simulink model "SIM_NonlinearPIwAW_2017b"  (R2017b)
settings: Solver=FixedStepAuto  StartTime=0.0  StopTime=9*0.25  FixedStep=h  RelTol=1e-3
values from neighbouring files (symbols this model uses):
  h = 1e-5    (= 1e-05)    [init.m]
  J = [0 -1; 1 0]    [generate_EKF.m]    (also in init.m)
  log_ts = 1e-5    (= 1e-05)    [init.m]
  lut_fr =     [friction.mat]
  omegam_ref = 157    [init.m]
  p = 2    [generate_EKF.m]
  P_init_dist = W_dist_noise    [init.m]
  pmsm_sew =     [config.mat]
  Psi_jac = [0.121, 0; 0, 0.0769]    [init.m]
  rsm_za =     [config.mat]
  SysConfig_SamplingTimeA = 0.00025    [config.mat]
  SysConfig_SamplingTimeB = 0.00025    [config.mat]
  u_DC = 556    [init.m]
  V_dist_noise = diag([2e0, 2e0])    [init.m]
  W_dist_noise = diag([1e-2, 1e-2, 1e4, 1e4])    [init.m]
  x_e_init_dist = zeros(4,1)    [init.m]
undefined symbols (not defined in the file or in its folder): DiscIntNeverNeededParam, f_pwm, k_i, k_p_tilde, uhat
libraries: simulink x4
(part 2 of 2)

== system SIM_NonlinearPIwAW_2017b/RSM_Control/Linear MPC/steady-state input computation ==
  psisk_ref : Inport
  wk : Inport  Port=2
  dist_est : Inport  Port=3
  Gain3 : Gain  Gain=J  Multiplication=Matrix(K*u)
  Gain4 : Gain  Gain=rsm_za.Rs
  Matrix Multiply : Product  Multiplication=Matrix(*)
  Product1 : Product
  Sum3 : Sum  Inputs=|++
  Sum4 : Sum  Inputs=|+-
  Unit Delay1 : UnitDelay  InitialCondition=[0,0]  SampleTime=-1
  Unit Delay2 : UnitDelay  InitialCondition=[0]  SampleTime=-1
  Unit Delay3 : UnitDelay  InitialCondition=[0,0]  SampleTime=-1
  inverse of dPsi/di : Constant  Value=inv(Psi_jac)
  u_ref : Outport
  wires:
  Sum3/1 -> u_ref/1
  dist_est/1 -> Unit Delay3/1
  Gain3/1 -> Product1/1
  psisk_ref/1 -> Gain3/1, Unit Delay1/1
  wk/1 -> Unit Delay2/1
  Matrix Multiply/1 -> Gain4/1
  Sum4/1 -> Sum3/2
  Gain4/1 -> Sum4/1
  Product1/1 -> Sum3/1
  Unit Delay1/1 -> Matrix Multiply/2
  Unit Delay2/1 -> Product1/2
  Unit Delay3/1 -> Sum4/2
  inverse of dPsi/di/1 -> Matrix Multiply/1

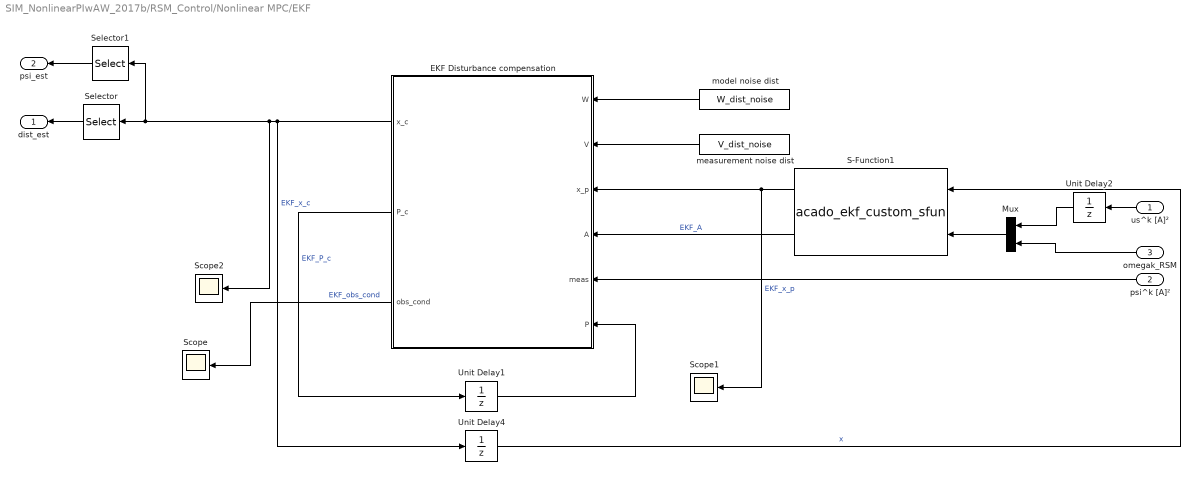
== system SIM_NonlinearPIwAW_2017b/RSM_Control/Nonlinear MPC/EKF  ==
  us^k [A]² : Inport
  psi^k [A]² : Inport  Port=2
  omegak_RSM : Inport  Port=3
  EKF Disturbance compensation : MATLAB Function  TreatAsAtomicUnit=on
  Mux : Mux  Inputs=2
  S-Function1 : S-Function  FunctionName=acado_ekf_custom_sfun  Parameters=[0 0 0 0]  SFunctionDeploymentMode=off  EnableBusSupport=off
  Scope : Scope
  Scope1 : Scope
  Scope2 : Scope
  Selector : Selector  InputPortWidth=4  IndexOptions=Index vector (dialog)  Indices=[3 4]  OutputSizes=1
  Selector1 : Selector  InputPortWidth=4  IndexOptions=Index vector (dialog)  Indices=[1 2]  OutputSizes=1
  Unit Delay1 : UnitDelay  InitialCondition=P_init_dist  SampleTime=-1
  Unit Delay2 : UnitDelay  InitialCondition=[0,0]  SampleTime=-1
  Unit Delay4 : UnitDelay  InitialCondition=x_e_init_dist  SampleTime=-1
  measurement noise dist : Constant  Value=V_dist_noise
  model noise dist : Constant  Value=W_dist_noise
  dist_est : Outport
  psi_est : Outport  Port=2
  wires:
  EKF Disturbance compensation/2(P_c) -> Unit Delay1/1  "EKF_P_c"
  measurement noise dist/1 -> EKF Disturbance compensation/2(V)
  EKF Disturbance compensation/3(obs_cond) -> Scope/1  "EKF_obs_cond"
  model noise dist/1 -> EKF Disturbance compensation/1(W)
  Unit Delay4/1 -> S-Function1/1  "x"
  EKF Disturbance compensation/1(x_c) -> Selector1/1, Selector/1, Scope2/1, Unit Delay4/1  "EKF_x_c"
  Unit Delay1/1 -> EKF Disturbance compensation/6(P)
  S-Function1/2 -> EKF Disturbance compensation/4(A)  "EKF_A"
  S-Function1/1 -> Scope1/1, EKF Disturbance compensation/3(x_p)  "EKF_x_p"
  psi^k [A]²/1 -> EKF Disturbance compensation/5(meas)
  Selector/1 -> dist_est/1
  us^k [A]²/1 -> Unit Delay2/1
  omegak_RSM/1 -> Mux/2
  Mux/1 -> S-Function1/2
  Selector1/1 -> psi_est/1
  Unit Delay2/1 -> Mux/1

== system SIM_NonlinearPIwAW_2017b/RSM_Control/Nonlinear MPC/steady-state input computation ==
  psisk_ref : Inport
  wk : Inport  Port=2
  dist_est : Inport  Port=3
  Gain3 : Gain  Gain=J  Multiplication=Matrix(K*u)
  Gain4 : Gain  Gain=rsm_za.Rs
  Product1 : Product
  S-Function : S-Function  FunctionName=acados_algebraic_solver_sfun  SFunctionDeploymentMode=off  EnableBusSupport=off
  Sum3 : Sum  Inputs=|++
  Sum4 : Sum  Inputs=|+-
  Unit Delay1 : UnitDelay  InitialCondition=[0,0]  SampleTime=-1
  Unit Delay2 : UnitDelay  InitialCondition=[0]  SampleTime=-1
  Unit Delay3 : UnitDelay  InitialCondition=[0,0]  SampleTime=-1
  u_ref : Outport
  wires:
  Sum3/1 -> u_ref/1
  dist_est/1 -> Unit Delay3/1
  Gain3/1 -> Product1/1
  psisk_ref/1 -> Gain3/1, Unit Delay1/1
  wk/1 -> Unit Delay2/1
  S-Function/1 -> Gain4/1
  Sum4/1 -> Sum3/2
  Gain4/1 -> Sum4/1
  Product1/1 -> Sum3/1
  Unit Delay1/1 -> S-Function/1
  Unit Delay2/1 -> Product1/2
  Unit Delay3/1 -> Sum4/2

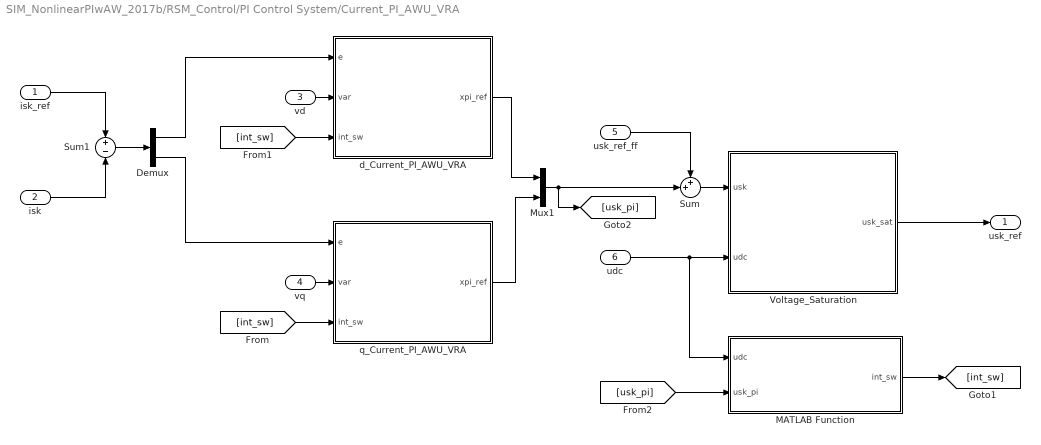
== system SIM_NonlinearPIwAW_2017b/RSM_Control/PI Control System/Current_PI_AWU_VRA ==
  isk_ref : Inport
  isk : Inport  Port=2
  vd : Inport  Port=3
  vq : Inport  Port=4
  usk_ref_ff : Inport  Port=5
  udc : Inport  Port=6
  Demux : Demux  Outputs=2
  MATLAB Function : MATLAB Function  TreatAsAtomicUnit=on
  Mux1 : Mux  Inputs=2
  Sum : Sum  Inputs=++|
  Sum1 : Sum  Inputs=+|-
  Voltage_Saturation : MATLAB Function  TreatAsAtomicUnit=on
  d_Current_PI_AWU_VRA : Subsystem  mask{VR=VRD, TN=TND}
      mask prompts: VR "Constant part of Proportional Gain K_p"; TN "Time Constant T_I"
      mask DialogControl DescGroupVar Prompt: Description
      mask DialogControl DescTextVar Prompt: PI-current controller with anti windup and parameter adaption.
  q_Current_PI_AWU_VRA : Subsystem  mask{VR=VRQ, TN=TNQ}
      mask prompts: VR "Constant part of Proportional Gain K_p"; TN "Time Constant T_I"
      mask DialogControl DescGroupVar Prompt: Description
      mask DialogControl DescTextVar Prompt: PI-current controller with anti windup and parameter adaption.
  usk_ref : Outport
  wires:
  Sum1/1 -> Demux/1
  isk/1 -> Sum1/2
  isk_ref/1 -> Sum1/1
  vq/1 -> q_Current_PI_AWU_VRA/2(var)
  [int_sw] -> d_Current_PI_AWU_VRA/3(int_sw)
  Demux/1 -> d_Current_PI_AWU_VRA/1(e)
  Sum/1 -> Voltage_Saturation/1(usk)
  q_Current_PI_AWU_VRA/1(xpi_ref) -> Mux1/2
  usk_ref_ff/1 -> Sum/1
  Mux1/1 -> [usk_pi], Sum/2
  Voltage_Saturation/1(usk_sat) -> usk_ref/1
  [int_sw] -> q_Current_PI_AWU_VRA/3(int_sw)
  d_Current_PI_AWU_VRA/1(xpi_ref) -> Mux1/1
  vd/1 -> d_Current_PI_AWU_VRA/2(var)
  Demux/2 -> q_Current_PI_AWU_VRA/1(e)
  udc/1 -> MATLAB Function/1(udc), Voltage_Saturation/2(udc)
  [usk_pi] -> MATLAB Function/2(usk_pi)
  MATLAB Function/1(int_sw) -> [int_sw]

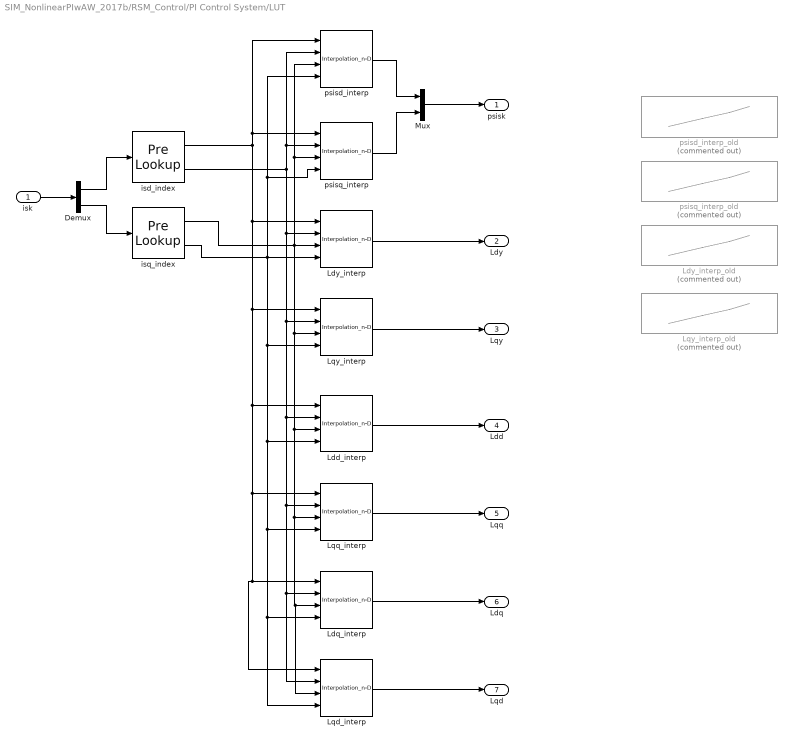
== system SIM_NonlinearPIwAW_2017b/RSM_Control/PI Control System/LUT ==
  isk : Inport
  Demux : Demux  Outputs=2
  Ldd_interp : Interpolation_n-D  Table=rsm_za.Ls.dd'  ExtrapMethod=Clip  InternalRulePriority=Speed
  Ldq_interp : Interpolation_n-D  Table=rsm_za.Ls.dq'  ExtrapMethod=Clip  InternalRulePriority=Speed
  Ldy_interp : Interpolation_n-D  Table=rsm_za.Ls.dy'  ExtrapMethod=Clip  InternalRulePriority=Speed
  Ldy_interp_old : Lookup_n-D  Commented=on  BreakpointsForDimension1=rsm_za.Is.d(1,:)  BreakpointsForDimension2=rsm_za.Is.q(:,1)  UseOneInputPortForAllInputData=on  Table=rsm_za.Ls.dy'  InternalRulePriority=Speed  RndMeth=Simplest  InputSameDT=on
  Lqd_interp : Interpolation_n-D  Table=rsm_za.Ls.qd'  ExtrapMethod=Clip  InternalRulePriority=Speed
  Lqq_interp : Interpolation_n-D  Table=rsm_za.Ls.qq'  ExtrapMethod=Clip  InternalRulePriority=Speed
  Lqy_interp : Interpolation_n-D  Table=rsm_za.Ls.qy'  ExtrapMethod=Clip  InternalRulePriority=Speed
  Lqy_interp_old : Lookup_n-D  Commented=on  BreakpointsForDimension1=rsm_za.Is.d(1,:)  BreakpointsForDimension2=rsm_za.Is.q(:,1)  UseOneInputPortForAllInputData=on  Table=rsm_za.Ls.qy'  InternalRulePriority=Speed  RndMeth=Simplest  InputSameDT=on
  Mux : Mux  Inputs=2
  isd_index : PreLookup  BreakpointsData=rsm_za.Is.d(1,:)  BeginIndexSearchUsingPreviousIndexResult=on  ExtrapMethod=Linear
  isq_index : PreLookup  BreakpointsData=rsm_za.Is.q(:,1)  BeginIndexSearchUsingPreviousIndexResult=on  ExtrapMethod=Linear
  psisd_interp : Interpolation_n-D  Table=rsm_za.Psis.d'  ExtrapMethod=Clip  InternalRulePriority=Speed
  psisd_interp_old : Lookup_n-D  Commented=on  BreakpointsForDimension1=rsm_za.Is.d(1,:)  BreakpointsForDimension2=rsm_za.Is.q(:,1)  UseOneInputPortForAllInputData=on  Table=rsm_za.Psis.d'  InternalRulePriority=Speed  RndMeth=Simplest  InputSameDT=on
  psisq_interp : Interpolation_n-D  Table=rsm_za.Psis.q'  ExtrapMethod=Clip  InternalRulePriority=Speed
  psisq_interp_old : Lookup_n-D  Commented=on  BreakpointsForDimension1=rsm_za.Is.d(1,:)  BreakpointsForDimension2=rsm_za.Is.q(:,1)  UseOneInputPortForAllInputData=on  Table=rsm_za.Psis.q'  InternalRulePriority=Speed  RndMeth=Simplest  InputSameDT=on
  psisk : Outport
  Ldy : Outport  Port=2
  Lqy : Outport  Port=3
  Ldd : Outport  Port=4
  Lqq : Outport  Port=5
  Ldq : Outport  Port=6
  Lqd : Outport  Port=7
  wires:
  psisd_interp/1 -> Mux/1
  psisq_interp/1 -> Mux/2
  Mux/1 -> psisk/1
  Ldy_interp/1 -> Ldy/1
  Lqy_interp/1 -> Lqy/1
  isk/1 -> Demux/1
  Demux/1 -> isd_index/1
  Demux/2 -> isq_index/1
  isd_index/1 -> Ldq_interp/1, Lqd_interp/1, Lqq_interp/1, Ldd_interp/1, Lqy_interp/1, Ldy_interp/1, psisq_interp/1, psisd_interp/1
  isd_index/2 -> Ldy_interp/2, Lqd_interp/2, Ldq_interp/2, Lqq_interp/2, Ldd_interp/2, Lqy_interp/2, psisd_interp/2, psisq_interp/2
  isq_index/1 -> Lqd_interp/3, Ldq_interp/3, Lqq_interp/3, Ldd_interp/3, Lqy_interp/3, psisd_interp/3, psisq_interp/3, Ldy_interp/3
  isq_index/2 -> psisq_interp/4, psisd_interp/4, Lqd_interp/4, Ldq_interp/4, Lqq_interp/4, Ldd_interp/4, Lqy_interp/4, Ldy_interp/4
  Ldq_interp/1 -> Ldq/1
  Lqq_interp/1 -> Lqq/1
  Ldd_interp/1 -> Ldd/1
  Lqd_interp/1 -> Lqd/1

== system SIM_NonlinearPIwAW_2017b/RSM_Control/PI Control System/Current_PI_AWU_VRA/d_Current_PI_AWU_VRA ==
  e : Inport
  var : Inport  Port=2
  int_sw : Inport  Port=3
  1/Tn : Gain  Gain=1/TN
  Constant : Constant  Value=0
  Discrete-Time Integrator : DiscreteIntegrator  SampleTime=-1  ICPrevOutput=DiscIntNeverNeededParam  ICPrevScaledInput=DiscIntNeverNeededParam
  Product1 : Product
  Sum : Sum  Inputs=|++
  Switch : Switch  Criteria=u2 > Threshold
  VR : Gain  Gain=VR
  xpi_ref : Outport
  wires:
  VR/1 -> Product1/2, 1/Tn/1
  Product1/1 -> Sum/1
  Discrete-Time Integrator/1 -> Sum/2
  Constant/1 -> Switch/3
  Sum/1 -> xpi_ref/1
  int_sw/1 -> Switch/2
  Switch/1 -> Discrete-Time Integrator/1
  1/Tn/1 -> Switch/1
  e/1 -> VR/1
  var/1 -> Product1/1

== system SIM_NonlinearPIwAW_2017b/RSM_Control/PI Control System/Current_PI_AWU_VRA/q_Current_PI_AWU_VRA ==
  e : Inport
  var : Inport  Port=2
  int_sw : Inport  Port=3
  1/Tn : Gain  Gain=1/TN
  Constant : Constant  Value=0
  Discrete-Time Integrator : DiscreteIntegrator  SampleTime=-1  ICPrevOutput=DiscIntNeverNeededParam  ICPrevScaledInput=DiscIntNeverNeededParam
  Product1 : Product
  Sum : Sum  Inputs=|++
  Switch : Switch  Criteria=u2 > Threshold
  VR : Gain  Gain=VR
  xpi_ref : Outport
  wires:
  var/1 -> Product1/1
  e/1 -> VR/1
  1/Tn/1 -> Switch/1
  Switch/1 -> Discrete-Time Integrator/1
  int_sw/1 -> Switch/2
  Sum/1 -> xpi_ref/1
  Constant/1 -> Switch/3
  Discrete-Time Integrator/1 -> Sum/2
  Product1/1 -> Sum/1
  VR/1 -> 1/Tn/1, Product1/2

== matlab function SIM_NonlinearPIwAW_2017b/PMSM_Control/ITP1 ==
  data: xs input; xk output; phik input
function xk = fcn(xs, phik)

    xk = [cos(phik), sin(phik); -sin(phik) cos(phik)]*xs;

== matlab function SIM_NonlinearPIwAW_2017b/PMSM_Control/TP1 ==
  data: xk input; xs output; phik input
function xs = fcn(xk, phik)

    xs = [cos(phik), -sin(phik); sin(phik) cos(phik)]*xk;

== matlab function SIM_NonlinearPIwAW_2017b/PMSM_Control/2L_SVM/2L_SVM ==
  data: sv0 output; uab_ref input size=2; udc input; svp output; svq output; t0 output; tp output; tq output; TPWM parameter; N parameter
function [sv0, svp, svq, t0, tp, tq] = nl_modulator( uab_ref, udc, TPWM, N)
%% N-Level space vector modulation
%  This block produces the switching times and vectors for an N-level VSI.

%% Calculate phase and angle of reference voltage vector

% Magnitude and angle
ang_uab_ref = atan2(uab_ref(2), uab_ref(1));

% 60° cosy
Ts = 2/3*udc/(N-1)*[1 0.5; 0 sqrt(3)/2];
Tsi = 1/(2/3*udc/(N-1))*[1 -sqrt(3)/3; 0 2/3*sqrt(3)]; 
Tp = @(phi) [cos(phi), sin(phi); -sin(phi) cos(phi)];
Hexs = [1, 0, -1, -1,  0,  1, 0;
        0, 1,  1,  0, -1, -1, 0];

%% Find 2-level sector and base vectors
tl_sec = 1 + floor(mod(ang_uab_ref, 2*pi)/ (pi/3));


%% Find sector and map reference to new subhexagon

% Transform alpha/beta voltage reference to 60° cosy
umn_ref = Tsi * uab_ref;

% Build subhexagon around rounded value of umn_ref and reduce valid roots
% to the inner vertices only -> (different approach to minimum distance to
% reference value approach)
Umn_hex_root = [round(umn_ref),round(umn_ref),round(umn_ref),round(umn_ref),round(umn_ref),round(umn_ref),round(umn_ref)];
Umn_hex_full = Umn_hex_root + Hexs;
 
idx = vectorNorm(Ts*Umn_hex_full) == min(vectorNorm(Ts*Umn_hex_full));
Umn_hex_inner = Umn_hex_full(:,idx);

% Among the remaining vertices, select candidate with minimum distance to
% the reference value as root vertex of the 2-level modulation subhexagon
idx = vectorNorm(Ts*Umn_hex_inner-uab_ref) == min(vectorNorm(Ts*Umn_hex_inner-uab_ref));
umn_root = Umn_hex_inner(:, idx); 

% Map reference voltage to subhexagon and transform back to alpha/beta cosy
umn_map = umn_ref - umn_root;
uab_map = Ts * umn_map;


%% Switching vector of subhexagon (mapping) -->  Table II in Shiny (2011)
if tl_sec < 3
    sv_hex = [umn_root(1) + umn_root(2), umn_root(2), 0]; 
elseif tl_sec < 5
    sv_hex = [0, -umn_root(1), -umn_root(1)-umn_root(2)];
else
    sv_hex = [umn_root(1), 0, -umn_root(2)];
end


%% Perform standard 2-level SVM on mapped voltage
ang_uab_map = atan2(uab_map(2), uab_map(1));
tl_map_sec = 1 + floor( mod(ang_uab_map, 2*pi) / (pi/3));

% Rotate vector to first sector and read-off vector portions
rpq = Tsi*Tp(pi/3*(tl_map_sec-1))*uab_map;
r0 = 1-rpq(1)-rpq(2);

switch tl_map_sec
    
    case 1
        svp_map = [1,0,0];
        svq_map = [1,1,0];
    case 2
        svp_map = [1,1,0];
        svq_map = [0,1,0];
    case 3
        svp_map = [0,1,0];
        svq_map = [0,1,1];
    case 4
        svp_map = [0,1,1];
        svq_map = [0,0,1];
    case 5 
        svp_map = [0,0,1];
        svq_map = [1,0,1];
    otherwise
        svp_map = [1,0,1];
        svq_map = [1,0,0];
end

tp = rpq(1)*TPWM;
tq = rpq(2)*TPWM;
t0 = r0*TPWM;

sv0 = sv_hex;
svp = svp_map + sv_hex;
svq = svq_map + sv_hex;

end

function [y] = vectorNorm(x)

    [m,n] = size(x);
    y = zeros(1, n);
    
    for i=1:n
        y(i) = sqrt(x(1,i)^2+x(2,i)^2);
    end

end

== matlab function SIM_NonlinearPIwAW_2017b/PMSM_Control/CurrentFeedForward_PMSM ==
  data: isk input; omegak input; usk_ref_ff output; pmsm_sew parameter
function usk_ref_ff  = fcn(isk, omegak, pmsm_sew)

    usk_ref_ff = omegak*[0 -1; 1 0]*([pmsm_sew.PsiPM; 0] + isk*pmsm_sew.Ls);

== matlab function SIM_NonlinearPIwAW_2017b/PMSM_Control/CurrentPIAWU/Voltage_Saturation ==
  data: usk input size=[2;1]; usk_sat output; udc input; int_sw output
function [usk_sat, int_sw] = voltage_saturation(usk, udc)

    usk_hat = sqrt(usk(1)^2+usk(2)^2);
    
    if usk_hat > udc/sqrt(3)
        
        int_sw = 0;
        usk_sat_hat = udc/sqrt(3);
        
    else 
        
        int_sw = 1;
        usk_sat_hat = usk_hat;
        
    end
    
    if usk_hat == 0
        usk_sat = [0;0];
    else
        usk_sat = usk_sat_hat / usk_hat * usk;
    end

== matlab function SIM_NonlinearPIwAW_2017b/2L_VSI_PMSM/NL_VSI/NL_VSI ==
  settings: updateMethod=DISCRETE
  data: sv0 input; svp input; svq input; t0 input; tp input; tq input; uabc0 output; udc input; TPWM parameter; HSIM parameter; N parameter; INT_OFFSET parameter; ucm output
  events: sw_int output FUNCTION_CALL_EVENT
function [uabc0, ucm]     = nl_vsi(sv0, svp, svq, t0, tp, tq, udc, TPWM, HSIM, N, INT_OFFSET)

persistent z;
persistent sv01_active sv02_active svp_active svq_active t0_active tp_active tq_active;

if isempty(z), z = 0; end
if isempty(sv01_active), sv01_active = [0,0,0]; end
if isempty(sv02_active), sv02_active = [1,1,1]; end
if isempty(svp_active), svp_active = [0,0,0]; end
if isempty(svq_active), svq_active = [0,0,0]; end
if isempty(t0_active), t0_active = 0; end
if isempty(tp_active), tp_active = 0; end
if isempty(tq_active), tq_active = 0; end

% Switching levels
SL = linspace(0, udc, N);

% Sample new data
if z==0
    sv01_active = sv0;              % First zero vector
    sv02_active = sv0 + [1,1,1];    % Second zero vector
    svp_active = svp;               % First adjacent vector
    svq_active = svq;               % Second adjacent vector
    t0_active = t0;                 % Zero vector cycle time
    tp_active = tp;                 % Vector one cycle time
    tq_active = tq;                 % Vector two cycle time
end

% Produce vector sequence (symmetrical)
if z < (t0_active/4)/HSIM
    sv_out = sv01_active;
elseif z < (t0_active/4 + tp_active/2)/HSIM
    sv_out = svp_active;
elseif z < (t0_active/4 + tp_active/2 + tq_active/2)/HSIM
    sv_out = svq_active;
elseif z < (t0_active*3/4 + tp_active/2 + tq_active/2)/HSIM
    sv_out = sv02_active;
elseif z < (t0_active*3/4 + tp_active/2 + tq_active)/HSIM
    sv_out = svq_active;
elseif z < (t0_active*3/4 + tp_active + tq_active)/HSIM
    sv_out = svp_active;
else
    sv_out = sv01_active;
end

% Create output
uabc0 = [SL(sv_out(1)+1);
         SL(sv_out(2)+1);
         SL(sv_out(3)+1)];
     
ucm = -1/3*(uabc0(1)+uabc0(2)+uabc0(3));

% Increase timer and reset if limit is reached
if z < (TPWM/HSIM)-1
    z = z+1;
else
  %  disp(['Time: ',num2str(2*t0+tp,tq,2),'\n']);
    z = 0;
end

% Trigger control (software interrupt) at specified time
if z == INT_OFFSET
    sw_int();
end

== matlab function SIM_NonlinearPIwAW_2017b/RSM_Control/PI Control System/Current_PI_AWU_VRA/MATLAB Function ==
  data: udc input; int_sw output; usk_pi input
function int_sw = fcn(udc, usk_pi)

    if usk_pi(1)^2+usk_pi(2)^2 > udc^2/3
        int_sw = 0;
    else
        int_sw = 1;
    end

== matlab function SIM_NonlinearPIwAW_2017b/RSM_Control/PI Control System/Current_PI_AWU_VRA/Voltage_Saturation ==
  data: usk input size=[2;1]; usk_sat output; udc input
function usk_sat  = voltage_saturation(usk, udc)

    usk_hat = sqrt(usk(1)^2+usk(2)^2);
    
    if usk_hat > udc/sqrt(3)
        
        usk_sat_hat = udc/sqrt(3);
        
    else 
        
        usk_sat_hat = usk_hat;
        
    end
    
    if usk_hat == 0
        usk_sat = [0;0];
    else
        usk_sat = usk_sat_hat / usk_hat * usk;
    end

== matlab function SIM_NonlinearPIwAW_2017b/RSM_Control/Nonlinear MPC/EKF /EKF Disturbance compensation ==
  data: W input; V input; x_p input; A input; meas input; x_c output; P_c output; P input; obs_cond output
function [x_c, P_c, obs_cond] = ExtendedKalmanFilterLoadDist(W, V, x_p, A, meas, P)
%#codegen

% EKF without torque measurements
% % Prediction step
% P_p = A*P*A.' + W;
% 
% % corrector step
% 
% % Kalman gain matrix
% C = [   1 0 0 0; ...
%         0 1 0 0];
%     
% K = P_p*C.'/(C*P_p*C.' + V);
% 
% x_c = x_p + K*(meas - C*x_p);
%     
% % A posteriori prediction error covariance
% P_c = (eye(4) - K*C)*P_p;
% 
% Om = [C; C*A; C*A^2; C*A^3];
% obs_cond = cond(Om);

% Prediction step
P_p = A*P*A.' + W;

% corrector step

% Kalman gain matrix
C = [   1 0 0 0; ...
        0 1 0 0];
    
K = P_p*C.'/(C*P_p*C.' + V);

x_c = x_p + K*(meas - C*x_p);
    
% A posteriori prediction error covariance
P_c = (eye(4) - K*C)*P_p;

Om = [C; C*A; C*A^2; C*A^3];
obs_cond = cond(Om);

end

== matlab function SIM_NonlinearPIwAW_2017b/RSM_Control/Nonlinear MPC/MATLAB Function ==
  data: isk input; psisd output; rsm_za parameter; psisq output
function [psisd, psisq] = fcn(isk, rsm_za)

    psisd = interp2(rsm_za.Is.d(1,:), rsm_za.Is.q(:,1), rsm_za.Psis.d, isk(1), isk(2), 'linear');
    psisq = interp2(rsm_za.Is.d(1,:), rsm_za.Is.q(:,1), rsm_za.Psis.q, isk(1), isk(2), 'linear');
    %Ldy = interp2(rsm_za.Is.d(1,:), rsm_za.Is.q(:,1), rsm_za.Ls.dy, isk(1), isk(2), 'linear');
   % Lqy = interp2(rsm_za.Is.d(1,:), rsm_za.Is.q(:,1), rsm_za.Ls.qy, isk(1), isk(2), 'linear');

== matlab function SIM_NonlinearPIwAW_2017b/2L_VSI_IM/NL_VSI/NL_VSI ==
  settings: updateMethod=DISCRETE
  data: sv0 input size=[1,3]; svp input size=[1,3]; svq input size=[1,3]; t0 input size=1; tp input size=1; tq input size=1; uabc0 output size=3; udc input size=1; TPWM parameter size=1; HSIM parameter size=1; N parameter size=1; INT_OFFSET parameter size=1; ucm output size=1
  events: sw_int output FUNCTION_CALL_EVENT
function [uabc0, ucm]     = nl_vsi(sv0, svp, svq, t0, tp, tq, udc, TPWM, HSIM, N, INT_OFFSET)

persistent z;
persistent sv01_active sv02_active svp_active svq_active t0_active tp_active tq_active;

if isempty(z), z = 0; end
if isempty(sv01_active), sv01_active = [0,0,0]; end
if isempty(sv02_active), sv02_active = [1,1,1]; end
if isempty(svp_active), svp_active = [0,0,0]; end
if isempty(svq_active), svq_active = [0,0,0]; end
if isempty(t0_active), t0_active = 0; end
if isempty(tp_active), tp_active = 0; end
if isempty(tq_active), tq_active = 0; end

% Switching levels
SL = linspace(0, udc, N);

% Sample new data
if z==0
    sv01_active = sv0;              % First zero vector
    sv02_active = sv0 + [1,1,1];    % Second zero vector
    svp_active = svp;               % First adjacent vector
    svq_active = svq;               % Second adjacent vector
    t0_active = t0;                 % Zero vector cycle time
    tp_active = tp;                 % Vector one cycle time
    tq_active = tq;                 % Vector two cycle time
end

% Produce vector sequence (symmetrical)
if z < (t0_active/4)/HSIM
    sv_out = sv01_active;
elseif z < (t0_active/4 + tp_active/2)/HSIM
    sv_out = svp_active;
elseif z < (t0_active/4 + tp_active/2 + tq_active/2)/HSIM
    sv_out = svq_active;
elseif z < (t0_active*3/4 + tp_active/2 + tq_active/2)/HSIM
    sv_out = sv02_active;
elseif z < (t0_active*3/4 + tp_active/2 + tq_active)/HSIM
    sv_out = svq_active;
elseif z < (t0_active*3/4 + tp_active + tq_active)/HSIM
    sv_out = svp_active;
else
    sv_out = sv01_active;
end

% Create output
uabc0 = [SL(sv_out(1)+1);
         SL(sv_out(2)+1);
         SL(sv_out(3)+1)];
     
ucm = -1/3*(uabc0(1)+uabc0(2)+uabc0(3));

% Increase timer and reset if limit is reached
if z < (TPWM/HSIM)-1
    z = z+1;
else
  %  disp(['Time: ',num2str(2*t0+tp,tq,2),'\n']);
    z = 0;
end

% Trigger control (software interrupt) at specified time
if z == INT_OFFSET
    sw_int();
end

== matlab function SIM_NonlinearPIwAW_2017b/RSM_Control/2L_SVM/2L_SVM ==
  data: sv0 output; uab_ref input size=2; udc input; svp output; svq output; t0 output; tp output; tq output; TPWM parameter; N parameter
function [sv0, svp, svq, t0, tp, tq] = nl_modulator( uab_ref, udc, TPWM, N)
%% N-Level space vector modulation
%  This block produces the switching times and vectors for an N-level VSI.

%% Calculate phase and angle of reference voltage vector

% Magnitude and angle
ang_uab_ref = atan2(uab_ref(2), uab_ref(1));

% 60° cosy
Ts = 2/3*udc/(N-1)*[1 0.5; 0 sqrt(3)/2];
Tsi = 1/(2/3*udc/(N-1))*[1 -sqrt(3)/3; 0 2/3*sqrt(3)]; 
Tp = @(phi) [cos(phi), sin(phi); -sin(phi) cos(phi)];
Hexs = [1, 0, -1, -1,  0,  1, 0;
        0, 1,  1,  0, -1, -1, 0];

%% Find 2-level sector and base vectors
tl_sec = 1 + floor(mod(ang_uab_ref, 2*pi)/ (pi/3));


%% Find sector and map reference to new subhexagon

% Transform alpha/beta voltage reference to 60° cosy
umn_ref = Tsi * uab_ref;

% Build subhexagon around rounded value of umn_ref and reduce valid roots
% to the inner vertices only -> (different approach to minimum distance to
% reference value approach)
Umn_hex_root = [round(umn_ref),round(umn_ref),round(umn_ref),round(umn_ref),round(umn_ref),round(umn_ref),round(umn_ref)];
Umn_hex_full = Umn_hex_root + Hexs;
 
idx = vectorNorm(Ts*Umn_hex_full) == min(vectorNorm(Ts*Umn_hex_full));
Umn_hex_inner = Umn_hex_full(:,idx);

% Among the remaining vertices, select candidate with minimum distance to
% the reference value as root vertex of the 2-level modulation subhexagon
idx = vectorNorm(Ts*Umn_hex_inner-uab_ref) == min(vectorNorm(Ts*Umn_hex_inner-uab_ref));
umn_root = Umn_hex_inner(:, idx); 

% Map reference voltage to subhexagon and transform back to alpha/beta cosy
umn_map = umn_ref - umn_root;
uab_map = Ts * umn_map;


%% Switching vector of subhexagon (mapping) -->  Table II in Shiny (2011)
if tl_sec < 3
    sv_hex = [umn_root(1) + umn_root(2), umn_root(2), 0]; 
elseif tl_sec < 5
    sv_hex = [0, -umn_root(1), -umn_root(1)-umn_root(2)];
else
    sv_hex = [umn_root(1), 0, -umn_root(2)];
end


%% Perform standard 2-level SVM on mapped voltage
ang_uab_map = atan2(uab_map(2), uab_map(1));
tl_map_sec = 1 + floor( mod(ang_uab_map, 2*pi) / (pi/3));

% Rotate vector to first sector and read-off vector portions
rpq = Tsi*Tp(pi/3*(tl_map_sec-1))*uab_map;
r0 = 1-rpq(1)-rpq(2);

switch tl_map_sec
    
    case 1
        svp_map = [1,0,0];
        svq_map = [1,1,0];
    case 2
        svp_map = [1,1,0];
        svq_map = [0,1,0];
    case 3
        svp_map = [0,1,0];
        svq_map = [0,1,1];
    case 4
        svp_map = [0,1,1];
        svq_map = [0,0,1];
    case 5 
        svp_map = [0,0,1];
        svq_map = [1,0,1];
    otherwise
        svp_map = [1,0,1];
        svq_map = [1,0,0];
end

tp = rpq(1)*TPWM;
tq = rpq(2)*TPWM;
t0 = r0*TPWM;

sv0 = sv_hex;
svp = svp_map + sv_hex;
svq = svq_map + sv_hex;

end

function [y] = vectorNorm(x)

    [m,n] = size(x);
    y = zeros(1, n);
    
    for i=1:n
        y(i) = sqrt(x(1,i)^2+x(2,i)^2);
    end

end

== matlab function SIM_NonlinearPIwAW_2017b/RSM_Control/Nonlinear MPC/MATLAB Function1 ==
  data: isk input; psisd output; rsm_za parameter; psisq output
function [psisd, psisq] = fcn(isk, rsm_za)

    psisd = interp2(rsm_za.Is.d(1,:), rsm_za.Is.q(:,1), rsm_za.Psis.d, isk(1), isk(2), 'linear');
    psisq = interp2(rsm_za.Is.d(1,:), rsm_za.Is.q(:,1), rsm_za.Psis.q, isk(1), isk(2), 'linear');
    %Ldy = interp2(rsm_za.Is.d(1,:), rsm_za.Is.q(:,1), rsm_za.Ls.dy, isk(1), isk(2), 'linear');
   % Lqy = interp2(rsm_za.Is.d(1,:), rsm_za.Is.q(:,1), rsm_za.Ls.qy, isk(1), isk(2), 'linear');

== matlab function SIM_NonlinearPIwAW_2017b/RSM_Control/current_trajectory/REF_GEN ==
  data: ENABLE_FLAG input; mmref output; xvec input; active_flag output; SysConfig_SamplingTimeA parameter; duration input
function [mmref,active_flag] = fcn(ENABLE_FLAG, xvec, SysConfig_SamplingTimeA, duration)

persistent n;
persistent z;

if isempty(n),n=1;end
if isempty(z),z=1;end


if ENABLE_FLAG == 1
    
    if n <=length(xvec)
        
        mmref = xvec(n);
        active_flag = 1;
        
        if z >= duration/SysConfig_SamplingTimeA
            z=0;
            n = n+1;
        else
            z=z+1; 
        end
        
    else
        mmref = xvec(n);
        active_flag = 0;
    end
    
    
else
    mmref = 0;
    n = 1;
    z = 0;
    active_flag = 0;
end

== matlab function SIM_NonlinearPIwAW_2017b/PMSM_Control/current_trajectory/REF_GEN ==
  data: ENABLE_FLAG input; mmref output; xvec input; active_flag output; SysConfig_SamplingTimeA parameter; duration input
function [mmref,active_flag] = fcn(ENABLE_FLAG, xvec, SysConfig_SamplingTimeA, duration)

persistent n;
persistent z;

if isempty(n),n=1;end
if isempty(z),z=1;end


if ENABLE_FLAG == 1
    
    if n <=length(xvec)
        
        mmref = xvec(n);
        active_flag = 1;
        
        if z >= duration/SysConfig_SamplingTimeA
            z=0;
            n = n+1;
        else
            z=z+1; 
        end
        
    else
        mmref = xvec(n);
        active_flag = 0;
    end
    
    
else
    mmref = 0;
    n = 1;
    z = 0;
    active_flag = 0;
end

== matlab function SIM_NonlinearPIwAW_2017b/RSM_Control/Nonlinear MPC/TP1 ==
  data: xk input; xs output; phik input
function xs = fcn(xk, phik)

    xs = [cos(phik), -sin(phik); sin(phik) cos(phik)]*xk;

== matlab function SIM_NonlinearPIwAW_2017b/RSM_Control/Christoph's controler/MATLAB Function ==
  settings: updateMethod=DISCRETE
  data: uskref input; uskrefsat output; uhat parameter
function uskrefsat  = fcn(uskref, uhat)

    uskref_norm = sqrt(uskref(1)^2+uskref(2)^2);

    if uskref_norm <= uhat
        uskrefsat = uskref;
    else
        uskrefsat = uskref/uskref_norm*uhat;
    end

== matlab function SIM_NonlinearPIwAW_2017b/RSM_Control/Christoph's controler/Current_FeedForward_IPMSM_RSM_PMSM ==
  data: psisk input; omegak input; usk_ref_ff output
function usk_ref_ff  = fcn(psisk, omegak)

    usk_ref_ff = omegak*[0 -1; 1 0]*psisk;

== matlab function SIM_NonlinearPIwAW_2017b/RSM_Control/Linear MPC/EKF /EKF Disturbance compensation ==
  data: W input; V input; x_p input; A input; meas input; x_c output; P_c output; P input; obs_cond output
function [x_c, P_c, obs_cond] = ExtendedKalmanFilterLoadDist(W, V, x_p, A, meas, P)
%#codegen

% EKF without torque measurements
% % Prediction step
% P_p = A*P*A.' + W;
% 
% % corrector step
% 
% % Kalman gain matrix
% C = [   1 0 0 0; ...
%         0 1 0 0];
%     
% K = P_p*C.'/(C*P_p*C.' + V);
% 
% x_c = x_p + K*(meas - C*x_p);
%     
% % A posteriori prediction error covariance
% P_c = (eye(4) - K*C)*P_p;
% 
% Om = [C; C*A; C*A^2; C*A^3];
% obs_cond = cond(Om);

% Prediction step
P_p = A*P*A.' + W;

% corrector step

% Kalman gain matrix
C = [   1 0 0 0; ...
        0 1 0 0];
    
K = P_p*C.'/(C*P_p*C.' + V);

x_c = x_p + K*(meas - C*x_p);
    
% A posteriori prediction error covariance
P_c = (eye(4) - K*C)*P_p;

Om = [C; C*A; C*A^2; C*A^3];
obs_cond = cond(Om);

end

== matlab function SIM_NonlinearPIwAW_2017b/RSM_Control/ITP1 ==
  data: xs input; xk output; phik input
function xk = fcn(xs, phik)

    xk = [cos(phik), sin(phik); -sin(phik) cos(phik)]*xs;

== matlab function SIM_NonlinearPIwAW_2017b/RSM_Control/Linear MPC/MATLAB Function ==
  data: isk input; psisd output; rsm_za parameter; psisq output
function [psisd, psisq] = fcn(isk, rsm_za)

    psisd = interp2(rsm_za.Is.d(1,:), rsm_za.Is.q(:,1), rsm_za.Psis.d, isk(1), isk(2), 'linear');
    psisq = interp2(rsm_za.Is.d(1,:), rsm_za.Is.q(:,1), rsm_za.Psis.q, isk(1), isk(2), 'linear');
    %Ldy = interp2(rsm_za.Is.d(1,:), rsm_za.Is.q(:,1), rsm_za.Ls.dy, isk(1), isk(2), 'linear');
   % Lqy = interp2(rsm_za.Is.d(1,:), rsm_za.Is.q(:,1), rsm_za.Ls.qy, isk(1), isk(2), 'linear');

== matlab function SIM_NonlinearPIwAW_2017b/RSM_Control/Linear MPC/MATLAB Function1 ==
  data: isk input; psisd output; rsm_za parameter; psisq output
function [psisd, psisq] = fcn(isk, rsm_za)

    psisd = interp2(rsm_za.Is.d(1,:), rsm_za.Is.q(:,1), rsm_za.Psis.d, isk(1), isk(2), 'linear');
    psisq = interp2(rsm_za.Is.d(1,:), rsm_za.Is.q(:,1), rsm_za.Psis.q, isk(1), isk(2), 'linear');
    %Ldy = interp2(rsm_za.Is.d(1,:), rsm_za.Is.q(:,1), rsm_za.Ls.dy, isk(1), isk(2), 'linear');
   % Lqy = interp2(rsm_za.Is.d(1,:), rsm_za.Is.q(:,1), rsm_za.Ls.qy, isk(1), isk(2), 'linear');

== matlab function SIM_NonlinearPIwAW_2017b/RSM_Control/PI Control System/TP1 ==
  data: xk input; xs output; phik input
function xs = fcn(xk, phik)

    xs = [cos(phik), -sin(phik); sin(phik) cos(phik)]*xk;

== matlab function SIM_NonlinearPIwAW_2017b/RSM_Control/Linear MPC/TP1 ==
  data: xk input; xs output; phik input
function xs = fcn(xk, phik)

    xs = [cos(phik), -sin(phik); sin(phik) cos(phik)]*xk;

== matlab function SIM_NonlinearPIwAW_2017b/RSM_Control/current trajectory generator/REF_GEN ==
  data: id_vec input; isk_ref output; iq_vec input; duration input
function isk_ref  = fcn(id_vec, iq_vec, duration)

persistent n;
persistent z;

if isempty(n),n=1;end
if isempty(z),z=1;end

if n > length(id_vec)
    n = 1;
end

isk_ref = [id_vec(n), iq_vec(n)];

if z >= duration/0.000250
    z=0;
    n = n+1;
else
    z=z+1;
end


end

== matlab function SIM_NonlinearPIwAW_2017b/PMSM_Electrical_System ==
  settings: updateMethod=DISCRETE
  data: uss input size=2; iss input size=2; omegam input size=1; phim input; d_iss output size=2; RS parameter; LS parameter; NP parameter; PSIPM parameter size=1; mel output size=1
function [d_iss, mel] = fcn(uss, iss, omegam, phim, RS, LS, NP, PSIPM)
  
    
    J2 = [0 -1; 1 0];
    
    psiss = LS*iss + [cos(NP*phim)*PSIPM; sin(NP*phim)*PSIPM];
    
    d_iss = 1/LS * (uss - RS*iss - NP*omegam*J2*[cos(NP*phim)*PSIPM; sin(NP*phim)*PSIPM]);
    
    mel = 3/2*NP*iss'*J2*psiss;

== matlab function SIM_NonlinearPIwAW_2017b/Testbench_Mechanical_System_with_Friction ==
  data: mel_M1 input; d_omegam output; mel_M2 input; MFR_LUT parameter; mm output; omegam input; THETAM_M1 parameter; THETAM_M2 parameter; WFR_LUT parameter
function [d_omegam, mm] = fcn(mel_M1, mel_M2, MFR_LUT, omegam, THETAM_M1, THETAM_M2, WFR_LUT)

    mfr = interp1(WFR_LUT, MFR_LUT, omegam, 'linear', 'extrap');
    mm = mel_M1 + mel_M2 + mfr;
    
    d_omegam = 1/(THETAM_M1 + THETAM_M2) * mm;

== matlab function SIM_NonlinearPIwAW_2017b/RSM_Control/PI Control System/Current_FeedForward_RSM_with_cross- coupling ==
  data: usdq_old input size=2; isdq input size=2; psisdq input size=2; omegak input size=1; usdq_ref_ff output size=2; Lsd input size=1; Lsq input size=1; Lsdq input size=1; Lsqd input; RS parameter size=1
function usdq_ref_ff  = fcn(usdq_old, isdq, psisdq, omegak, Lsd, Lsq, Lsdq, Lsqd, RS)

    % Ysdq = Lsdq^-1 = Ysdq_si + Ysdq_de = [Ysd_si  0     ] + [0        Ysm_de]
    %                                      [0       Ysq_si]   [Ysm_de   0     ]
    %
    % Ys = Ysdq_si^-1*Ysdq_de
    Ys = [0 -Lsdq./Lsq; -Lsqd./Lsd, 0];

    usdq_ref_ff = - (  -omegak*[0 -1; 1 0]*psisdq + ...
                        Ys*(usdq_old-RS*isdq-omegak*[0 -1; 1 0]*psisdq));

== matlab function SIM_NonlinearPIwAW_2017b/RSM_Electrical_System ==
  settings: updateMethod=DISCRETE
  data: uss input size=2; psiss input size=2; phim input; d_psiss output size=2; iss output size=2; RS parameter; NP parameter; ISD parameter; mel output size=1; ISQ parameter; PSISD parameter; PSISQ parameter; isk output; psisk output
function [d_psiss, iss, mel, isk, psisk] = fcn(uss, psiss, phim, RS, NP, ISD, ISQ, PSISD, PSISQ)
  
    
    J2 = [0 -1; 1 0];
    TP = [cos(NP*phim) -sin(NP*phim); sin(NP*phim) cos(NP*phim)];
    ITP = [cos(NP*phim) sin(NP*phim); -sin(NP*phim) cos(NP*phim)];
    
    psisk = ITP*psiss;
    isk = bilinearInverse2DInterp(psisk, ISD, ISQ, PSISD, PSISQ);
    
    iss = TP*isk;
    d_psiss = uss - RS*iss;
    
    mel = 3/2*NP*iss'*J2*psiss;
    
end


function isk = bilinearInverse2DInterp(psisk, ISD, ISQ, PSISD, PSISQ)

    %% Interval finding algorithm (by Peter Landsmann)
    %Searching Index Interval
    [~, n] = size(PSISD);
    FLAG_ixf = 0;
    ixd0 = round(n/2);
    ixq0 = ixd0;
    ixd1 = ixd0 + 1;
    ixq1 = ixq0 + 1;
    psi00 = [0 0]';
    psi01 = [0 0]';
    psi10 = [0 0]';
    psi11 = [0 0]';

    while FLAG_ixf<2                                                           % Stop when interval is found
        FLAG_ixf = 0;
        ixd1 = ixd0 + 1;
        ixq1 = ixq0 + 1;

        % Define vertices
        psi00 = [PSISD(ixq0,ixd0) PSISQ(ixq0,ixd0)]';
        psi01 = [PSISD(ixq0,ixd1) PSISQ(ixq0,ixd1)]';
        psi10 = [PSISD(ixq1,ixd0) PSISQ(ixq1,ixd0)]';
        psi11 = [PSISD(ixq1,ixd1) PSISQ(ixq1,ixd1)]';

        % d-axis search (left/right)

        % Reference is located left of the quad (if a Psi plane is considered -> straight line)
        if psisk(1) < psi00(1) + (psi10(1)-psi00(1))/(psi10(2)-psi00(2))*(psisk(2)-psi00(2))
            if ixd0>1                                                      % If inside limits
                ixd0 = ixd0 - 1;
            else
                FLAG_ixf = 1;
            end

        % Reference is located right of the quad
        elseif psisk(1) > psi01(1) + (psi11(1)-psi01(1))/(psi11(2)-psi01(2))*(psisk(2)-psi01(2))
            if ixd1 < n               
                ixd0 = ixd0 + 1;
            else
                FLAG_ixf = 1;
            end

        % Reference is located neither left nor right of the quad => Interval
        % found
        else
            FLAG_ixf = 1;
        end

        % q-axis search (top/bottom)

        % Reference is located below the quad
        if     psisk(2) < psi00(2) + (psi01(2)-psi00(2))/(psi01(1)-psi00(1))*(psisk(1)-psi00(1))
            if ixq0>1                              
                ixq0 = ixq0 - 1;
            else
                FLAG_ixf = FLAG_ixf + 1;
            end

        % Reference is located above the quad
        elseif psisk(2) > psi10(2) + (psi11(2) - psi10(2))/(psi11(1) - psi10(1))*(psisk(1)-psi10(1))
            if ixq1 < n
                ixq0 = ixq0 + 1;
            else
                FLAG_ixf = FLAG_ixf + 1;
            end

        % Reference is located neither above nor below the quad => Interval
        % found
        else
            FLAG_ixf = FLAG_ixf + 1;
        end
    end
    
    %% Bilinear inverse interpolation (http://www.iquilezles.org/www/articles/ibilinear/ibilinear.htm)
    ixdq = [ixd0, ixq0, ixd1, ixq1];
    
    %   10 ------- Q --- 11
    %    |         |      |
    %    |         *      |
    %    |         |      |
    %   00 ------- P --- 01

    %    P = Psi00 + u(Psi01-Psi00)
    %    Q = Psi10 + u(Psi11-Psi10)
    % Psi* = P+v(Q-P)
    % => X = Psi*-Psi00 = A*u + B*v + C*u*v
    % 
    % Eliminate u => quadratic polynomial => find v (0..1) => calculate u
    % (0..1)

    % Define intermediate variables
    X = psisk-psi00;
    A = psi01-psi00;
    B = psi10-psi00;
    C = psi11-psi10-psi01+psi00;

    % Define coeffecients of quadratic equation
    c2 = X(2)*A(1)-X(1)*A(2);
    c1 = X(2)*C(1)-X(1)*C(2)+B(1)*A(2)-B(2)*A(1);
    c0 = B(1)*C(2)-B(2)*C(1);

    % Solve quadratic equation
    v1 = (-c1+sqrt(c1^2-4*c0*c2))/(2*c0);
    v2 = (-c1-sqrt(c1^2-4*c0*c2))/(2*c0);

    % Pick the solution, which is element of [0,1]
    v=0;
    if (v1>=0 && v1 <= 1), v = v1; end
    if (v2>=0 && v2 <= 1), v = v2; end

    % Determine the second interpolation parameter
    u = (X(1)-B(1)*v)/(A(1)+C(1)*v);

    % Interpolation of the output
    isk = [ISD(1,ixdq(1)) + u*(ISD(1,ixdq(3)) - ISD(1,ixdq(1))); ...
           ISQ(ixdq(2),1) + v*(ISQ(ixdq(4),1) - ISQ(ixdq(2),1))];
end
